simulink model "fishball_qam16"  (R2026a)
settings: Solver=FixedStepDiscrete  StopTime=inf
model workspace (MAT data in the model file):
  refC = [-0.948683298051+0.948683298051i; -0.948683298051+0.316227766017i; -0.948683298051-0.948683298051i; -0.948683298051-0.316227766017i; -0.316227766017+0.948683298051i; -0.316227766017+0.316227766017i; -0.316227766017-0.948683298051i; -0.316227766017-0.316227766017i; 0.948683298051+0.948683298051i; 0.948683298051+0.316227766017i; 0.948683298051-0.948683298051i; 0.948683298051-0.316227766017i; 0.316227766017+0.948683298051i; 0.316227766017+0.316227766017i; 0.316227766017-0.948683298051i; 0.316227766017-0.316227766017i]
  txWave = [-0.202903178541+0.429447828746i -0.00458403585636+0.485334679149i 0.226537966315+0.548477583559i 0.420020157686+0.575133777949i 0.510506741751+0.516442493559i 0.47231157613+0.340724077006i 0.349300905787+0.109854617859i 0.212288944929-0.0954046910109i 0.122952807318-0.199957041169i 0.104778596294-0.169894631233i 0.135205128669-0.0549137143799i 0.166737377368+0.0805679215738i ... (4096 elements, 4096x1)]
libraries: commsync2 x2, commrfcorlib x1, commfilt2 x1
settings Model: Creator=matthieu  LastModifiedBy=matthieu

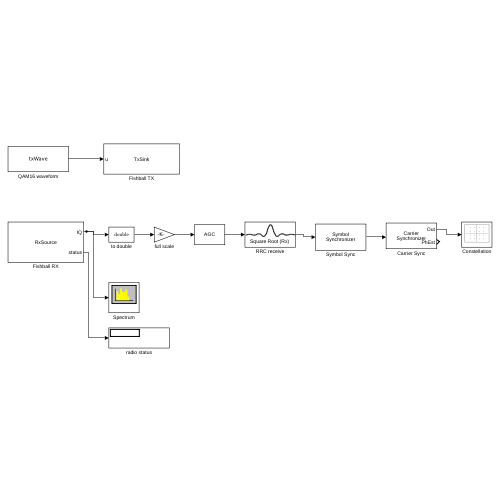
[thumbnail: Simulink's stored preview of the top-level diagram]
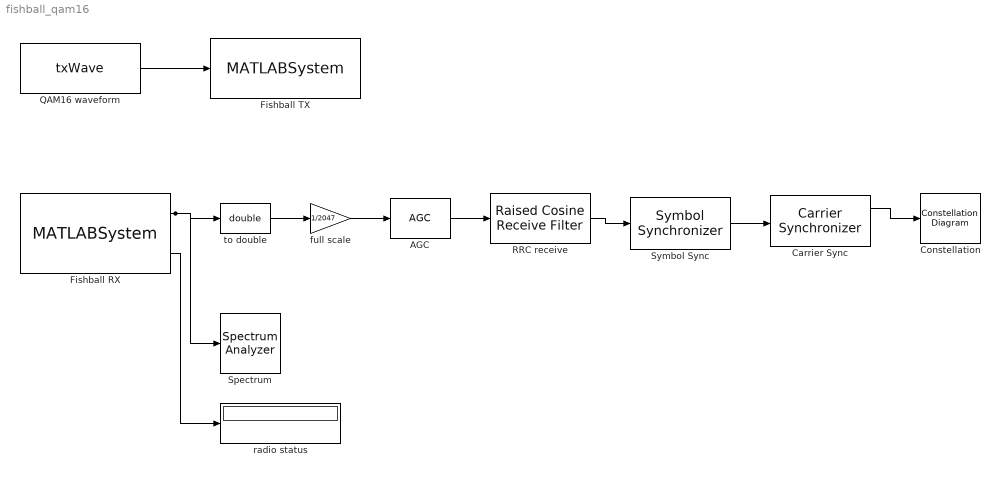
== system fishball_qam16 ==
  AGC : commrfcorlib/AGC  LegacyMode=off  DetectorMethod=Rectifier  LoopMethod=Linear  UpdatePeriod=100  StepSize=0.1  AdaptationStepSize=0.01  DesiredOutputPower=1  AveragingLength=100  MaximumGain=30  MaxPowerGain=60  GainOutputPort=off  InputPowerOutputPort=off  SimulateUsing=Interpreted execution
  Carrier Sync : commsync2/Carrier Synchronizer  Modulation=QAM  ModulationPhaseOffset=Auto  CustomPhaseOffset=0  SamplesPerSymbol=1  DampingFactor=0.707  NormalizedLoopBandwidth=0.01  EstimatedPhaseErrorOutputPort=on  SimulateUsing=Code generation
  Constellation : ConstellationDiagram  ReferenceConstellation=refC
  Fishball RX : MATLABSystem  System=fishball.RxSource  ChannelMapping=RX1  CenterFrequency=900000000  RFBandwidth=4608000  RFPort=A Balanced  GainSource=Manual  Gain=20  BasebandSampleRate=2304000  FabricDecimation=1  SamplesPerFrame=4096  EnableQuadratureTracking=on  EnableRFDCTracking=on  EnableBasebandDCTracking=on  EnableRxFIR=off  ControlPorts=none  StatusUpdatePeriod=1  SimulateUsing=Interpreted execution
      mask Type: fishball.RxSource
  Fishball TX : MATLABSystem  System=fishball.TxSink  ChannelMapping=TX1  CenterFrequency=900000000  Gain=-30  PadDb=20  Headroom=10  BasebandSampleRate=2304000  SamplesPerFrame=4096  Cyclic=on  SampleGpio=off  SimulateUsing=Interpreted execution
      mask Type: fishball.TxSink
  QAM16 waveform : Constant  Value=txWave  SampleTime=0.00177777777778
  RRC receive : commfilt2/Raised Cosine Receive Filter  filtType=Square root  R=0.35  filtSpan=10  N=4  downFactor=2  downOffset=0  filterGain=1  InputProcessing=Columns as channels (frame based)  RateOptions=Enforce single-rate processing  framing=Mute  checkCoeff=off  variableName=rcRxFilt  currentFiltSpan=10  D=5  inputOffset=0  sampMode=Mute  saveAsFlag=0  rateMode=Downsampling  checkGain=Normalized  launchFVT=on  roundingMode=Floor  overflowMode=off  coeffDataTypeStr=Inherit: Same word length as input  coeffMin=[]  coeffMax=[]  coeffLastDataTypeStr=Inherit: Same word length as input  accumDataTypeStr=Inherit: Same as product output  accumLastDataTypeStr=Inherit: Same as product output  outputDataTypeStr=Inherit: Same as accumulator  outputMin=[]  outputMax=[]  outputLastDataTypeStr=Inherit: Same as accumulator
  Spectrum : SpectrumAnalyzer  WindowInvariantSamplesPerUpdate=on
  Symbol Sync : commsync2/Symbol Synchronizer  Modulation=PAM/PSK/QAM  TimingErrorDetector=Gardner (non-data-aided)  SamplesPerSymbol=2  DampingFactor=1  NormalizedLoopBandwidth=0.01  DetectorGain=2.7  TimingErrorOutputPort=off  SimulateUsing=Code generation
  full scale : Gain  Gain=1/2047
  radio status : Display
  to double : DataTypeConversion  OutDataTypeStr=double  SaturateOnIntegerOverflow=off  RndMeth=Floor
  wires:
  QAM16 waveform/1 -> Fishball TX/1
  Fishball RX/1 -> to double/1, Spectrum/1
  to double/1 -> full scale/1
  full scale/1 -> AGC/1
  AGC/1 -> RRC receive/1
  RRC receive/1 -> Symbol Sync/1
  Symbol Sync/1 -> Carrier Sync/1
  Carrier Sync/1 -> Constellation/1
  Fishball RX/2 -> radio status/1
